simulink model "impulse_input_sec_ord"  (R2024b)
settings: Solver=VariableStepAuto  StartTime=0.0  StopTime=10.0  RelTol=1e-3
settings Model: Creator=darkk157night  LastModifiedBy=darkk157night

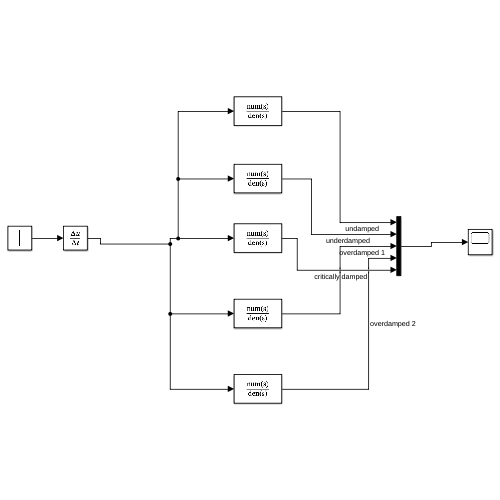
[thumbnail: Simulink's stored preview of the top-level diagram]
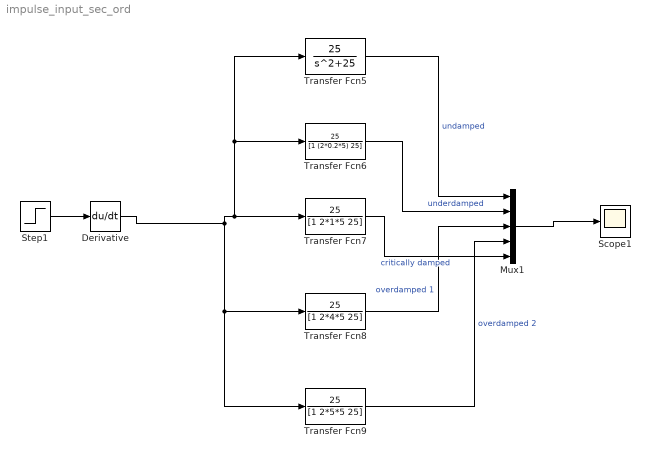
== system impulse_input_sec_ord ==
  Derivative : Derivative
  Mux1 : Mux  Inputs=5
  Scope1 : Scope
  Step1 : Step  SampleTime=0
  Transfer Fcn5 : TransferFcn  Numerator=[25]  Denominator=[1 0 25]
  Transfer Fcn6 : TransferFcn  Numerator=[25]  Denominator=[1 (2*0.2*5) 25]
  Transfer Fcn7 : TransferFcn  Numerator=[25]  Denominator=[1 2*1*5 25]
  Transfer Fcn8 : TransferFcn  Numerator=[25]  Denominator=[1 2*4*5 25]
  Transfer Fcn9 : TransferFcn  Numerator=[25]  Denominator=[1 2*5*5 25]
  wires:
  Mux1/1 -> Scope1/1
  Transfer Fcn5/1 -> Mux1/1  "undamped"
  Transfer Fcn7/1 -> Mux1/5  "critically damped"
  Step1/1 -> Derivative/1
  Transfer Fcn8/1 -> Mux1/3  "overdamped 1"
  Transfer Fcn6/1 -> Mux1/2  "underdamped"
  Derivative/1 -> Transfer Fcn5/1, Transfer Fcn6/1, Transfer Fcn7/1, Transfer Fcn9/1, Transfer Fcn8/1
  Transfer Fcn9/1 -> Mux1/4  "overdamped 2"
